simulink model "sim"  (R2017a)
settings: Solver=ode45  StartTime=0.0  StopTime=5000.0  RelTol=1e-3
settings Model: Creator=dvl  LastModifiedBy=dvl

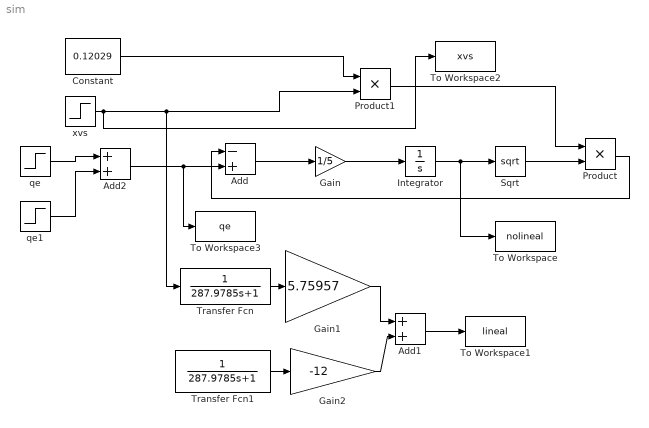
== system sim ==
  Add : Sum  Inputs=-+
  Add1 : Sum
  Add2 : Sum
  Constant : Constant  Value=0.12029
  Gain : Gain  Gain=1/5
  Gain1 : Gain  Gain=5.75957
  Gain2 : Gain  Gain=-12
  Integrator : Integrator
  Product : Product
  Product1 : Product
  Sqrt : Sqrt  SaturateOnIntegerOverflow=on
  To Workspace : ToWorkspace  VariableName=nolineal  SaveFormat=Timeseries  SampleTime=-1
  To Workspace1 : ToWorkspace  VariableName=lineal  SaveFormat=Timeseries  SampleTime=-1
  To Workspace2 : ToWorkspace  VariableName=xvs  SaveFormat=Timeseries  SampleTime=-1
  To Workspace3 : ToWorkspace  VariableName=qe  SaveFormat=Timeseries  SampleTime=-1
  Transfer Fcn : TransferFcn  Denominator=[287.9785 1]
  Transfer Fcn1 : TransferFcn  Denominator=[287.9785 1]
  qe : Step  Time=0  After=0.1042  SampleTime=0
  qe1 : Step  Time=2000  After=-0.01042  SampleTime=0
  xvs : Step  Time=4000  Before=0.5  After=0.495  SampleTime=0
  wires:
  Add/1 -> Gain/1
  Gain/1 -> Integrator/1
  Integrator/1 -> To Workspace/1, Sqrt/1
  Constant/1 -> Product1/1
  Product1/1 -> Product/1
  Sqrt/1 -> Product/2
  Product/1 -> Add/1
  xvs/1 -> To Workspace2/1, Product1/2, Transfer Fcn/1
  Gain1/1 -> Add1/1
  Gain2/1 -> Add1/2
  Transfer Fcn/1 -> Gain1/1
  Transfer Fcn1/1 -> Gain2/1
  Add1/1 -> To Workspace1/1
  qe/1 -> Add2/1
  qe1/1 -> Add2/2
  Add2/1 -> To Workspace3/1, Add/2
